simulink model "BMS_MainStateMachine_COM_Harness_MIL"  (R2022b)
settings: configuration reference "BMS_Sw_CodeGenConfig" (kept outside this file)
model workspace (MAT data in the model file):
  BATT.Manufacturer = 'Panasonic'
  BATT.Chemistry = 'Lithium Ion'
  BATT.Model = 'UR18650ZTA'
  BATT.Diameter = 18.2399997711
  BATT.Length = 65.0999984741
  BATT.CycleLife = 500
  BATT.Package.Ns_Module = 1
  BATT.Package.NumModules = 3
  BATT.Capacity.Rate = 2.84999990463
  BATT.Capacity.Min = 2.90000009537
  BATT.Capacity.Max = 3.09999990463
  BATT.Capacity.MaxQ = 3.30460000038
  BATT.Capacity.Type = 3
  BATT.Res.R0 = 0.0113329999149
  BATT.Res.R1 = 0.00999999977648
  BATT.Res.C1 = 0.00300000002608
  BATT.Res.R0_EOL = 0.0142999999225
  BATT.Res.lambda = 1.06599998474
  BATT.Voltage.Nominal = 3.70000004768
  BATT.Voltage.NominalVolt = 3.40000009537
  BATT.Voltage.Cut_off = 3
  BATT.Voltage.Init_Dchrg = 3.38000011444
  BATT.Voltage.Full_Dchrg = 4.19999980927
  BATT.Voltage.Max_Chrg = 4.34999990463
  BATT.Voltage.Over = 4.40000009537
  BATT.Voltage.Under = 3
  BATT.Voltage.threshold = 0.5
  BATT.Voltage.V_LUT = [3 3.09999990463 3.20000004768 3.29999995232 3.40000009537 3.5 3.59999990463 3.70000004768 3.79999995232 3.90000009537 4 4.09999990463 4.19999980927]
  BATT.Temperature.Max = 50
  BATT.Temperature.Min = -20
  BATT.Temperature.Nominal = 20
  BATT.Temperature.dQ_dt = 0.00499999988824
  BATT.Temperature.T_LUT = [-20 -15 -10 -5 0 5 10 15 20 25 30 35 40 45 50]
  BATT.Temperature.derate_Fact = [0.598999977112 0.69580000639 0.769999980927 0.824599981308 0.870000004768 0.912999987602 0.949999988079 0.981000006199 1 1.00499999523 1.00999999046 1.01800000668 1.02999997139 1.05700004101 1.10000002384]
  BATT.Current.Dchrg = 6
  BATT.Current.Chrg = 1.45000004768
  BATT.Current.Chrgfast = 2.5
  BATT.Current.ChrgSafe = 0.0579999983311
  BATT.Current.Overthreshold = 0.20000000298
  BATT.Current.threshold = 0.00999999977648
  BATT.Current.CV_Gain = 20
  BATT.SoC.SoC0 = 50
  BATT.SoC.max = 100
  BATT.SoC.min = 0
  BATT.SoC.alpha = 0.25
  BATT.SoC.Values = [0 10 20 30 40 50 60 70 80 90 100]
  BATT.SoC.iter = 10
  BATT.SoC.TableData = [20 30 40 55 70 85 90 100 100 100 100 100 ... (195 elements, 13x15)]
  BATT.Balancing.Mode : BMS_BalMode_Enum (value not decoded)
  BATT.Balancing.ThresholdOn = 0.0250000003725
  BATT.Balancing.ThresholdOff = 0.00999999977648
  BATT.Balancing.BalWaitOff = 5
  BATT.Balancing.BalWaitOn = 10
  BATT.Balancing.Freq = 1000
  BATT.Balancing.Duty = 0.449999988079
  ChrgBit = Simulink.Parameter
  ChrgBit.Value = 0
  ChrgBit.Description = 'charger Fault Bit'
  ChrgBit.DataType = 'uint8'
  ChrgBit.Complexity = 'real'
  ChrgBit.Dimensions = [1 1]
  CntTime = Simulink.Parameter
  CntTime.Value = 500
  CntTime.Description = 'Conector waiting Time'
  CntTime.DataType = 'uint16'
  CntTime.Complexity = 'real'
  CntTime.Dimensions = [1 1]
  CntTimeout = Simulink.Parameter
  CntTimeout.Value = 5000
  CntTimeout.Description = 'Conector Timeout'
  CntTimeout.DataType = 'uint16'
  CntTimeout.Complexity = 'real'
  CntTimeout.Dimensions = [1 1]
  CurrTimeout = Simulink.Parameter
  CurrTimeout.Value = 1000
  CurrTimeout.Description = 'Over Current Timeout'
  CurrTimeout.DataType = 'uint16'
  CurrTimeout.Complexity = 'real'
  CurrTimeout.Dimensions = [1 1]
  FaultResetTime = Simulink.Parameter
  FaultResetTime.Value = 5000
  FaultResetTime.Description = 'Fault Reset waiting Time'
  FaultResetTime.DataType = 'uint16'
  FaultResetTime.Complexity = 'real'
  FaultResetTime.Dimensions = [1 1]
  HighTempBit = Simulink.Parameter
  HighTempBit.Value = 4
  HighTempBit.Description = 'High Temperature Bit'
  HighTempBit.DataType = 'uint8'
  HighTempBit.Complexity = 'real'
  HighTempBit.Dimensions = [1 1]
  InvrBit = Simulink.Parameter
  InvrBit.Value = 1
  InvrBit.Description = 'Inverter Fault Bit'
  InvrBit.DataType = 'uint8'
  InvrBit.Complexity = 'real'
  InvrBit.Dimensions = [1 1]
  LowTempBit = Simulink.Parameter
  LowTempBit.Value = 3
  LowTempBit.Description = 'Low Temperature Bit'
  LowTempBit.DataType = 'uint8'
  LowTempBit.Complexity = 'real'
  LowTempBit.Dimensions = [1 1]
  OverCurrBit = Simulink.Parameter
  OverCurrBit.Value = 2
  OverCurrBit.Description = 'Over Current Bit'
  OverCurrBit.DataType = 'uint8'
  OverCurrBit.Complexity = 'real'
  OverCurrBit.Dimensions = [1 1]
  OverVoltBit = Simulink.Parameter
  OverVoltBit.Value = 6
  OverVoltBit.Description = 'Over voltage Bit'
  OverVoltBit.DataType = 'uint8'
  OverVoltBit.Complexity = 'real'
  OverVoltBit.Dimensions = [1 1]
  Schedule.BMS_CurrentLimitsCalc_Task = 0.1
  Schedule.BMS_MainStateMachine_Task = 0.05
  Schedule.BMS_BalancingLogic_Task = 0.25
  Schedule.BMS_EstimateSOC_Task = 0.2
  Schedule.BMS_EstimateSOH_Task = 0.2
  TempTimeout = Simulink.Parameter
  TempTimeout.Value = 1000
  TempTimeout.Description = 'Teperature Timeout'
  TempTimeout.DataType = 'uint16'
  TempTimeout.Complexity = 'real'
  TempTimeout.Dimensions = [1 1]
  UnderVoltBit = Simulink.Parameter
  UnderVoltBit.Value = 5
  UnderVoltBit.Description = 'Under voltage Bit'
  UnderVoltBit.DataType = 'uint8'
  UnderVoltBit.Complexity = 'real'
  UnderVoltBit.Dimensions = [1 1]
  VoltSensBit = Simulink.Parameter
  VoltSensBit.Value = 7
  VoltSensBit.Description = 'Voltage sensing Bit'
  VoltSensBit.DataType = 'uint8'
  VoltSensBit.Complexity = 'real'
  VoltSensBit.Dimensions = [1 1]
settings Model: DataDictionary=BMS_Arch_DD.sldd  Creator=MAAM  LastModifiedBy=MAAM
settings ConfigSetRef: SourceName=BMS_Sw_CodeGenConfig

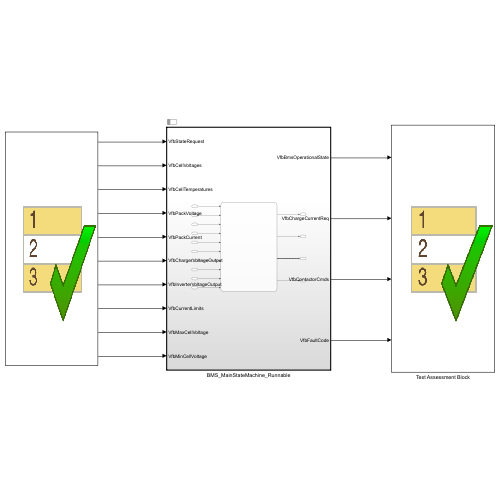
[thumbnail: Simulink's stored preview of the top-level diagram]
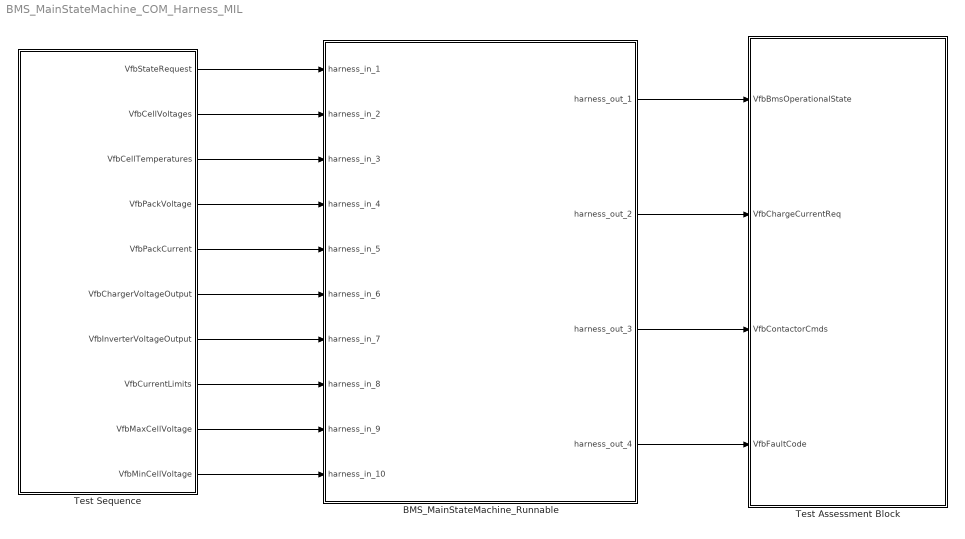
== system BMS_MainStateMachine_COM_Harness_MIL ==
  BMS_MainStateMachine_Runnable : Subsystem  Tag=__SL_testing_harness_stub_  Priority=1
  Test Assessment Block : Test Sequence  Tag=__SLT_ASMT__  TreatAsAtomicUnit=on
  Test Sequence : Test Sequence  TreatAsAtomicUnit=on
  wires:
  Test Sequence/3(VfbCellTemperatures) -> BMS_MainStateMachine_Runnable/3(harness_in_3)
  Test Sequence/4(VfbPackVoltage) -> BMS_MainStateMachine_Runnable/4(harness_in_4)
  Test Sequence/5(VfbPackCurrent) -> BMS_MainStateMachine_Runnable/5(harness_in_5)
  Test Sequence/6(VfbChargerVoltageOutput) -> BMS_MainStateMachine_Runnable/6(harness_in_6)
  Test Sequence/7(VfbInverterVoltageOutput) -> BMS_MainStateMachine_Runnable/7(harness_in_7)
  Test Sequence/8(VfbCurrentLimits) -> BMS_MainStateMachine_Runnable/8(harness_in_8)
  Test Sequence/9(VfbMaxCellVoltage) -> BMS_MainStateMachine_Runnable/9(harness_in_9)
  Test Sequence/10(VfbMinCellVoltage) -> BMS_MainStateMachine_Runnable/10(harness_in_10)
  Test Sequence/1(VfbStateRequest) -> BMS_MainStateMachine_Runnable/1(harness_in_1)
  Test Sequence/2(VfbCellVoltages) -> BMS_MainStateMachine_Runnable/2(harness_in_2)
  BMS_MainStateMachine_Runnable/1(harness_out_1) -> Test Assessment Block/1(VfbBmsOperationalState)
  BMS_MainStateMachine_Runnable/2(harness_out_2) -> Test Assessment Block/2(VfbChargeCurrentReq)
  BMS_MainStateMachine_Runnable/3(harness_out_3) -> Test Assessment Block/3(VfbContactorCmds)
  BMS_MainStateMachine_Runnable/4(harness_out_4) -> Test Assessment Block/4(VfbFaultCode)

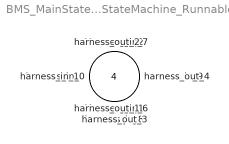
== system BMS_MainStateMachine_COM_Harness_MIL/BMS_MainStateMachine_Runnable ==
  harness_in_1 : Inport
  harness_in_2 : Inport  Port=2
  harness_in_3 : Inport  Port=3
  harness_in_4 : Inport  Port=4
  harness_in_5 : Inport  Port=5
  harness_in_6 : Inport  Port=6
  harness_in_7 : Inport  Port=7
  harness_in_8 : Inport  Port=8
  harness_in_9 : Inport  Port=9
  harness_in_10 : Inport  Port=10
  harness_out_1 : Outport
  harness_out_2 : Outport  Port=2
  harness_out_3 : Outport  Port=3
  harness_out_4 : Outport  Port=4

== stateflow chart BMS_MainStateMachine_COM_Harness_MIL/Test Assessment Block ==
  state Run
    state step_1_1
    state step_1_2
    (default) -> (junction 22)
    Run -> (junction 22)
    (junction 22) -> (junction 23) [order 1] : [t < 5
        | ]
    (junction 23) -> step_1_1 [order 1] : [~in(Run.step_1_1)]
    (junction 23) -> (junction 26) [order 2]
    (junction 31) -> (junction 32)
    (junction 32) -> step_1_2 [order 1] : [~in(Run.step_1_2)]
    (junction 32) -> (junction 35) [order 2]
    (junction 22) -> (junction 31) [order 2]
  (default) -> Run
  data: VfbBmsOperationalState input Enum: BMS_State_Enum size=[1]; VfbChargeCurrentReq input single size=[1]; VfbContactorCmds input Bus: BMS_strContactorCmds size=[1]; VfbFaultCode input uint8 size=[1]

== stateflow chart BMS_MainStateMachine_COM_Harness_MIL/Test Sequence ==
  settings: updateMethod=DISCRETE  sampleTime=0.05
  state Run
    %% Initialize data outputs.
    VfbStateRequest = BMS_State_Enum.BMS_Standby;
    VfbCellVoltages = single(zeros(3, 1));
    VfbCellTemperatures = single(zeros(3, 1));
    VfbPackVoltage = single(0);
    VfbPackCurrent = single(0);
    VfbChargerVoltageOutput = single(0);
    VfbInverterVoltageOutput = single(0);
    VfbCurrentLimits = single(zeros(2, 1));
    VfbMaxCellVoltage = single(0);
    VfbMinCellVoltage = single(0);
  (default) -> Run
  data: VfbStateRequest output Enum: BMS_State_Enum size=[1]; VfbCellVoltages output single size=[3]; VfbCellTemperatures output single size=[3]; VfbPackVoltage output single size=[1]; VfbPackCurrent output single size=[1]; VfbChargerVoltageOutput output single size=[1]; VfbInverterVoltageOutput output single size=[1]; VfbCurrentLimits output single size=[2]; VfbMaxCellVoltage output single size=[1]; VfbMinCellVoltage output single size=[1]
